simulink model "proyecto_automation"  (R2021a)
settings: Solver=VariableStepAuto  StartTime=0.0  StopTime=1900  RelTol=1e-3
values from neighbouring files (symbols this model uses):
  B = 0.029    [Parameters_setting.m]
  J = 0.1    [Parameters_setting.m]
  Ke = 0.6    [Parameters_setting.m]
  Kt = 0.6    [Parameters_setting.m]
  La = 1e-3    (= 0.001)    [Parameters_setting.m]
  Ra = 1    [Parameters_setting.m]
libraries: pid_lib x6, simulink x1
settings Model: Creator=csanc  LastModifiedBy=csanc

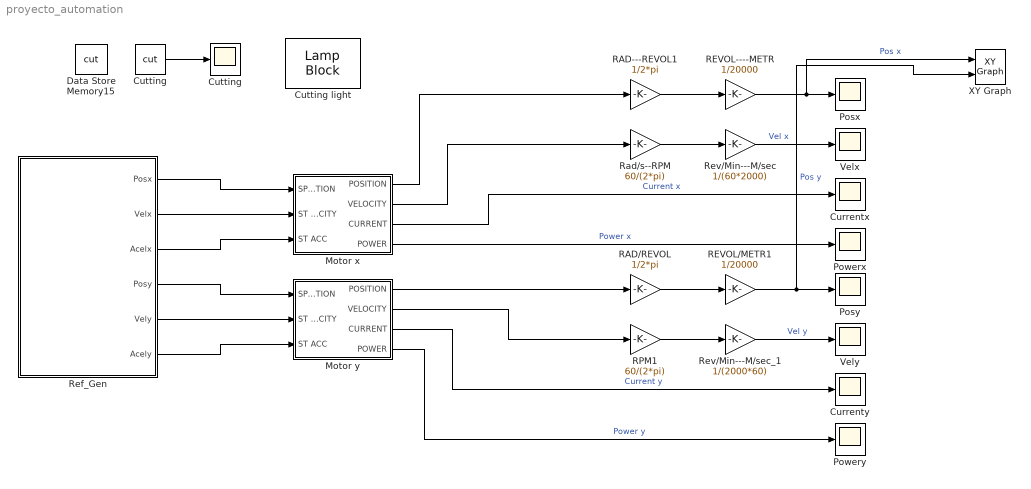
== system proyecto_automation ==
  Currentx : Scope
  Currenty : Scope
  Cutting : Scope
  "Cutting " : DataStoreRead  DataStoreName=cut  IndexOptions=Index vector (dialog)  Indices=1  OutputSizes=1
  Cutting light : LampBlock  Icon=LightingSwitch
  Data Store Memory15 : DataStoreMemory  DataStoreName=cut  ReadBeforeWriteMsg=warning  WriteAfterWriteMsg=warning  WriteAfterReadMsg=warning  ShowAdditionalParam=off
  Motor x : Subsystem
  Motor y : Subsystem
  Posx : Scope
  Posy : Scope
  Powerx : Scope
  Powery : Scope
  RAD---REVOL1 : Gain  Gain=1/2*pi
  RAD/REVOL : Gain  Gain=1/2*pi
  REVOL----METR : Gain  Gain=1/20000
  REVOL/METR1 : Gain  Gain=1/20000
  RPM1 : Gain  Gain=60/(2*pi)
  Rad/s--RPM : Gain  Gain=60/(2*pi)
  Ref_Gen : Subsystem
  Rev/Min---M/sec : Gain  Gain=1/(60*2000)
  Rev/Min---M/sec_1 : Gain  Gain=1/(2000*60)
  Velx : Scope
  Vely : Scope
  XY Graph : simulink/Sinks/XY Graph  xmin=0  xmax=3  ymin=0  ymax=2  st=1
  wires:
  Rad/s--RPM/1 -> Rev/Min---M/sec/1
  REVOL----METR/1 -> XY Graph/1, Posx/1  "Pos x"
  Rev/Min---M/sec/1 -> Velx/1  "Vel x"
  Ref_Gen/1(Posx) -> Motor x/1(SP POSITION)
  Ref_Gen/2(Velx) -> Motor x/2(ST VELOCITY)
  Ref_Gen/3(Acelx) -> Motor x/3(ST ACC)
  Motor x/2(VELOCITY) -> Rad/s--RPM/1
  Motor x/3(CURRENT) -> Currentx/1  "Current x"
  Motor x/4(POWER) -> Powerx/1  "Power x"
  Rev/Min---M/sec_1/1 -> Vely/1  "Vel y"
  REVOL/METR1/1 -> XY Graph/2, Posy/1  "Pos y"
  RAD/REVOL/1 -> REVOL/METR1/1
  RPM1/1 -> Rev/Min---M/sec_1/1
  Motor y/1(POSITION) -> RAD/REVOL/1
  Motor y/2(VELOCITY) -> RPM1/1
  Motor y/3(CURRENT) -> Currenty/1  "Current y"
  Motor y/4(POWER) -> Powery/1  "Power y"
  RAD---REVOL1/1 -> REVOL----METR/1
  Motor x/1(POSITION) -> RAD---REVOL1/1
  Ref_Gen/4(Posy) -> Motor y/1(SP POSITION)
  Ref_Gen/5(Vely) -> Motor y/2(ST VELOCITY)
  Ref_Gen/6(Acely) -> Motor y/3(ST ACC)
  "Cutting "/1 -> Cutting/1

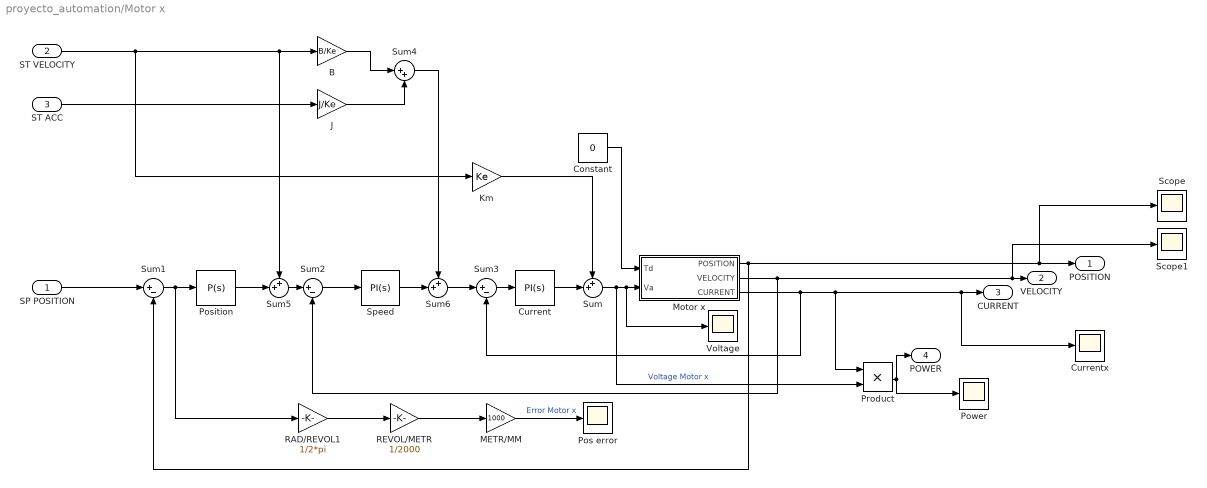
== system proyecto_automation/Motor x ==
  SP POSITION : Inport
  ST VELOCITY : Inport  Port=2
  ST ACC : Inport  Port=3
  B : Gain  Gain=B/Ke
  Constant : Constant  Value=0
  Current : pid_lib/PID Controller  Controller=PI  Form=Parallel  TimeDomain=Continuous-time  UseExternalTs=off  SampleTime=-1  IntegratorMethod=Forward Euler  FilterMethod=Forward Euler  ControllerParametersSource=internal  P=La*1000  I=Ra*1000  D=0  UseFilter=on  N=100  TunerSelectOption=Transfer Function Based (PID Tuner App)  InitialConditionSource=internal  InitialConditionForIntegrator=0  InitialConditionForFilter=0  DifferentiatorICPrevScaledInput=0  ExternalReset=none  TrackingMode=off  Kt=1  LimitOutput=off  SatLimitsSource=internal  UpperSaturationLimit=inf  LowerSaturationLimit=-inf  LinearizeAsGain=on  AntiWindupMode=none  Kb=1  POutMin=[]  POutMax=[]  IOutMin=[]  IOutMax=[]  DOutMin=[]  DOutMax=[]  NOutMin=[]  NOutMax=[]  SumOutMin=[]  SumOutMax=[]  SaturationOutMin=[]  SaturationOutMax=[]  PParamMin=[]  PParamMax=[]  IParamMin=[]  IParamMax=[]  DParamMin=[]  DParamMax=[]  NParamMin=[]  NParamMax=[]  KbParamMin=[]  KbParamMax=[]  KtParamMin=[]  KtParamMax=[]  KbOutMin=[]  KbOutMax=[]  KtOutMin=[]  KtOutMax=[]  IntegratorOutMin=[]  IntegratorOutMax=[]  FilterOutMin=[]  FilterOutMax=[]  SumI1OutMin=[]  SumI1OutMax=[]  SumI2OutMin=[]  SumI2OutMax=[]  SumI3OutMin=[]  SumI3OutMax=[]  SumI4OutMin=[]  SumI4OutMax=[]  SumDOutMin=[]  SumDOutMax=[]  DifferentiatorOutMin=[]  DifferentiatorOutMax=[]  FilterDiffOutCoefMin=[]  FilterDiffOutCoefMax=[]  ReciprocalOutMin=[]  ReciprocalOutMax=[]  SumDenOutMin=[]  SumDenOutMax=[]  SumNumOutMin=[]  SumNumOutMax=[]  DivideOutMin=[]  DivideOutMax=[]  UdiffTsProdOutMin=[]  UdiffTsProdOutMax=[]  NTsProdOutMin=[]  NTsProdOutMax=[]  UintegralTsProdOutMin=[]  UintegralTsProdOutMax=[]  UngainTsProdOutMin=[]  UngainTsProdOutMax=[]  IntegratorContinuousStateAttributes=''  IntegratorStateMustResolveToSignalObject=off  IntegratorRTWStateStorageClass=Auto  FilterContinuousStateAttributes=''  FilterStateMustResolveToSignalObject=off  FilterRTWStateStorageClass=Auto  ParallelPVariant=InternalParameters  IdealPVariant=Disabled  IVariant=InternalParameters  DVariant=Disabled  IntegratorVariant=Continuous  SatVariant=Disabled  AWVariant=Passthrough  PCopyVariant=Disabled  TRVariant=Disabled  FdbkBlocksVariant=Forward  IdealPFdbkVariant=Disabled  SatFdbkVariant=Disabled  DerivativeFilterVariant=Disabled  NVariant=Disabled  NCopyVariant=Disabled_SignalSpec  FilterICVariant=Disabled  IntegratorICVariant=InternalICs  ExternalResetVariant=Disabled  TRSumVariant=Passthrough  SumFdbkVariant=Disabled  SumVariant=Sum_PI  TsampFilterVariant=InternalTs  TsampNgainVariant=Passthrough  TsampIntegralVariant=Passthrough  ExternalSaturationOutDataTypeStr=Inherit: Same as second input
  Currentx : Scope
  J : Gain  Gain=J/Ke
  Km : Gain  Gain=Ke
  METR/MM : Gain  Gain=1000
  Motor x : Subsystem
  Pos error : Scope
  Position : pid_lib/PID Controller  Controller=P  Form=Parallel  TimeDomain=Continuous-time  UseExternalTs=on  SampleTime=-1  IntegratorMethod=Forward Euler  FilterMethod=Forward Euler  ControllerParametersSource=internal  P=1.1  I=1  D=0  UseFilter=on  N=100  TunerSelectOption=Transfer Function Based (PID Tuner App)  InitialConditionSource=internal  InitialConditionForIntegrator=0  InitialConditionForFilter=0  DifferentiatorICPrevScaledInput=0  ExternalReset=none  TrackingMode=off  Kt=1  LimitOutput=off  SatLimitsSource=internal  UpperSaturationLimit=inf  LowerSaturationLimit=-inf  LinearizeAsGain=on  AntiWindupMode=none  Kb=1  POutMin=[]  POutMax=[]  IOutMin=[]  IOutMax=[]  DOutMin=[]  DOutMax=[]  NOutMin=[]  NOutMax=[]  SumOutMin=[]  SumOutMax=[]  SaturationOutMin=[]  SaturationOutMax=[]  PParamMin=[]  PParamMax=[]  IParamMin=[]  IParamMax=[]  DParamMin=[]  DParamMax=[]  NParamMin=[]  NParamMax=[]  KbParamMin=[]  KbParamMax=[]  KtParamMin=[]  KtParamMax=[]  KbOutMin=[]  KbOutMax=[]  KtOutMin=[]  KtOutMax=[]  IntegratorOutMin=[]  IntegratorOutMax=[]  FilterOutMin=[]  FilterOutMax=[]  SumI1OutMin=[]  SumI1OutMax=[]  SumI2OutMin=[]  SumI2OutMax=[]  SumI3OutMin=[]  SumI3OutMax=[]  SumI4OutMin=[]  SumI4OutMax=[]  SumDOutMin=[]  SumDOutMax=[]  DifferentiatorOutMin=[]  DifferentiatorOutMax=[]  FilterDiffOutCoefMin=[]  FilterDiffOutCoefMax=[]  ReciprocalOutMin=[]  ReciprocalOutMax=[]  SumDenOutMin=[]  SumDenOutMax=[]  SumNumOutMin=[]  SumNumOutMax=[]  DivideOutMin=[]  DivideOutMax=[]  UdiffTsProdOutMin=[]  UdiffTsProdOutMax=[]  NTsProdOutMin=[]  NTsProdOutMax=[]  UintegralTsProdOutMin=[]  UintegralTsProdOutMax=[]  UngainTsProdOutMin=[]  UngainTsProdOutMax=[]  IntegratorContinuousStateAttributes=''  IntegratorStateMustResolveToSignalObject=off  IntegratorRTWStateStorageClass=Auto  FilterContinuousStateAttributes=''  FilterStateMustResolveToSignalObject=off  FilterRTWStateStorageClass=Auto  ParallelPVariant=InternalParameters  IdealPVariant=Disabled  IVariant=Disabled  DVariant=Disabled  IntegratorVariant=Disabled  SatVariant=Disabled  AWVariant=Disabled  PCopyVariant=Disabled  TRVariant=Disabled  FdbkBlocksVariant=Forward  IdealPFdbkVariant=Disabled  SatFdbkVariant=Disabled  DerivativeFilterVariant=Disabled  NVariant=Disabled  NCopyVariant=Disabled_SignalSpec  FilterICVariant=Disabled  IntegratorICVariant=Disabled  ExternalResetVariant=Disabled  TRSumVariant=Passthrough  SumFdbkVariant=Disabled  SumVariant=Passthrough_P  TsampFilterVariant=InternalTs  TsampNgainVariant=Passthrough  TsampIntegralVariant=Disabled_SignalSpec  ExternalSaturationOutDataTypeStr=Inherit: Same as second input
  Power : Scope
  Product : Product
  RAD/REVOL1 : Gain  Gain=1/2*pi
  REVOL/METR : Gain  Gain=1/2000
  Scope : Scope
  Scope1 : Scope
  Speed : pid_lib/PID Controller  Controller=PI  Form=Parallel  TimeDomain=Continuous-time  UseExternalTs=off  SampleTime=-1  IntegratorMethod=Forward Euler  FilterMethod=Forward Euler  ControllerParametersSource=internal  P=10*J  I=10*B  D=0  UseFilter=on  N=100  TunerSelectOption=Transfer Function Based (PID Tuner App)  InitialConditionSource=internal  InitialConditionForIntegrator=0  InitialConditionForFilter=0  DifferentiatorICPrevScaledInput=0  ExternalReset=none  TrackingMode=off  Kt=1  LimitOutput=off  SatLimitsSource=internal  UpperSaturationLimit=inf  LowerSaturationLimit=-inf  LinearizeAsGain=on  AntiWindupMode=none  Kb=1  POutMin=[]  POutMax=[]  IOutMin=[]  IOutMax=[]  DOutMin=[]  DOutMax=[]  NOutMin=[]  NOutMax=[]  SumOutMin=[]  SumOutMax=[]  SaturationOutMin=[]  SaturationOutMax=[]  PParamMin=[]  PParamMax=[]  IParamMin=[]  IParamMax=[]  DParamMin=[]  DParamMax=[]  NParamMin=[]  NParamMax=[]  KbParamMin=[]  KbParamMax=[]  KtParamMin=[]  KtParamMax=[]  KbOutMin=[]  KbOutMax=[]  KtOutMin=[]  KtOutMax=[]  IntegratorOutMin=[]  IntegratorOutMax=[]  FilterOutMin=[]  FilterOutMax=[]  SumI1OutMin=[]  SumI1OutMax=[]  SumI2OutMin=[]  SumI2OutMax=[]  SumI3OutMin=[]  SumI3OutMax=[]  SumI4OutMin=[]  SumI4OutMax=[]  SumDOutMin=[]  SumDOutMax=[]  DifferentiatorOutMin=[]  DifferentiatorOutMax=[]  FilterDiffOutCoefMin=[]  FilterDiffOutCoefMax=[]  ReciprocalOutMin=[]  ReciprocalOutMax=[]  SumDenOutMin=[]  SumDenOutMax=[]  SumNumOutMin=[]  SumNumOutMax=[]  DivideOutMin=[]  DivideOutMax=[]  UdiffTsProdOutMin=[]  UdiffTsProdOutMax=[]  NTsProdOutMin=[]  NTsProdOutMax=[]  UintegralTsProdOutMin=[]  UintegralTsProdOutMax=[]  UngainTsProdOutMin=[]  UngainTsProdOutMax=[]  IntegratorContinuousStateAttributes=''  IntegratorStateMustResolveToSignalObject=off  IntegratorRTWStateStorageClass=Auto  FilterContinuousStateAttributes=''  FilterStateMustResolveToSignalObject=off  FilterRTWStateStorageClass=Auto  ParallelPVariant=InternalParameters  IdealPVariant=Disabled  IVariant=InternalParameters  DVariant=Disabled  IntegratorVariant=Continuous  SatVariant=Disabled  AWVariant=Passthrough  PCopyVariant=Disabled  TRVariant=Disabled  FdbkBlocksVariant=Forward  IdealPFdbkVariant=Disabled  SatFdbkVariant=Disabled  DerivativeFilterVariant=Disabled  NVariant=Disabled  NCopyVariant=Disabled_SignalSpec  FilterICVariant=Disabled  IntegratorICVariant=InternalICs  ExternalResetVariant=Disabled  TRSumVariant=Passthrough  SumFdbkVariant=Disabled  SumVariant=Sum_PI  TsampFilterVariant=InternalTs  TsampNgainVariant=Passthrough  TsampIntegralVariant=Passthrough  ExternalSaturationOutDataTypeStr=Inherit: Same as second input
  Sum : Sum  Inputs=++|
  Sum1 : Sum  Inputs=|+-
  Sum2 : Sum  Inputs=|+-
  Sum3 : Sum  Inputs=|+-
  Sum4 : Sum  Inputs=|++
  Sum5 : Sum  Inputs=++|
  Sum6 : Sum  Inputs=++|
  Voltage : Scope
  POSITION : Outport
  VELOCITY : Outport  Port=2
  CURRENT : Outport  Port=3
  POWER : Outport  Port=4
  wires:
  Current/1 -> Sum/2
  ST VELOCITY/1 -> Km/1, Sum5/1, B/1
  Sum/1 -> Product/2, Voltage/1, Motor x/2(Va)  "Voltage Motor x"
  Sum2/1 -> Speed/1
  Motor x/2(VELOCITY) -> Sum2/2, Scope1/1, VELOCITY/1
  Motor x/3(CURRENT) -> Currentx/1, CURRENT/1, Product/1, Sum3/2
  J/1 -> Sum4/2
  Sum3/1 -> Current/1
  Sum1/1 -> RAD/REVOL1/1, Position/1
  ST ACC/1 -> J/1
  Motor x/1(POSITION) -> Scope/1, POSITION/1, Sum1/2
  Constant/1 -> Motor x/1(Td)
  B/1 -> Sum4/1
  Product/1 -> POWER/1, Power/1
  Position/1 -> Sum5/2
  Sum5/1 -> Sum2/1
  Sum6/1 -> Sum3/1
  Speed/1 -> Sum6/2
  SP POSITION/1 -> Sum1/1
  Km/1 -> Sum/1
  Sum4/1 -> Sum6/1
  RAD/REVOL1/1 -> REVOL/METR/1
  REVOL/METR/1 -> METR/MM/1
  METR/MM/1 -> Pos error/1  "Error Motor x"

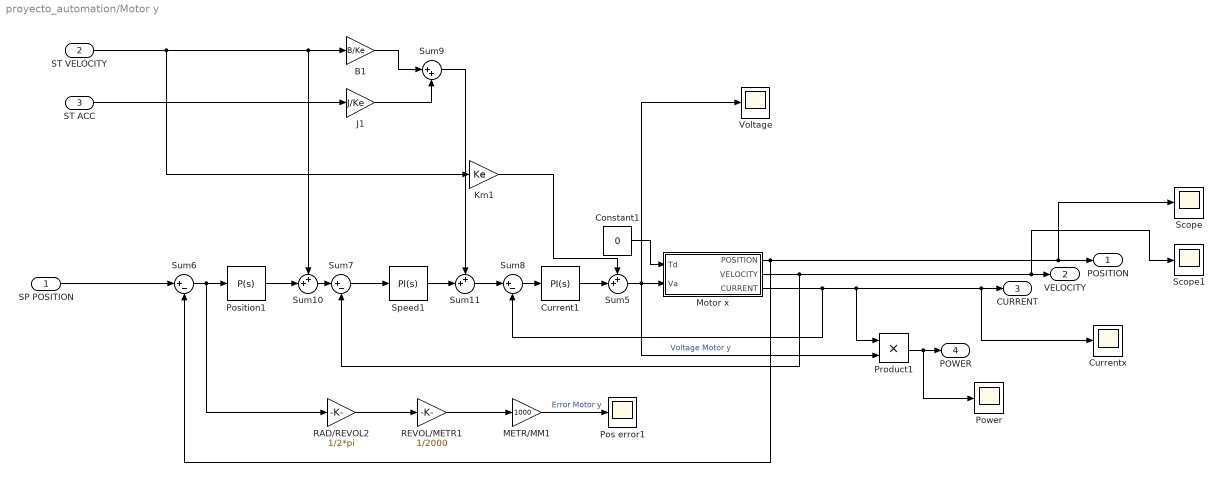
== system proyecto_automation/Motor y ==
  SP POSITION : Inport
  ST VELOCITY : Inport  Port=2
  ST ACC : Inport  Port=3
  B1 : Gain  Gain=B/Ke
  Constant1 : Constant  Value=0
  Current1 : pid_lib/PID Controller  Controller=PI  Form=Parallel  TimeDomain=Continuous-time  UseExternalTs=off  SampleTime=-1  IntegratorMethod=Forward Euler  FilterMethod=Forward Euler  ControllerParametersSource=internal  P=La*1000  I=Ra*1000  D=0  UseFilter=on  N=100  TunerSelectOption=Transfer Function Based (PID Tuner App)  InitialConditionSource=internal  InitialConditionForIntegrator=0  InitialConditionForFilter=0  DifferentiatorICPrevScaledInput=0  ExternalReset=none  TrackingMode=off  Kt=1  LimitOutput=off  SatLimitsSource=internal  UpperSaturationLimit=inf  LowerSaturationLimit=-inf  LinearizeAsGain=on  AntiWindupMode=none  Kb=1  POutMin=[]  POutMax=[]  IOutMin=[]  IOutMax=[]  DOutMin=[]  DOutMax=[]  NOutMin=[]  NOutMax=[]  SumOutMin=[]  SumOutMax=[]  SaturationOutMin=[]  SaturationOutMax=[]  PParamMin=[]  PParamMax=[]  IParamMin=[]  IParamMax=[]  DParamMin=[]  DParamMax=[]  NParamMin=[]  NParamMax=[]  KbParamMin=[]  KbParamMax=[]  KtParamMin=[]  KtParamMax=[]  KbOutMin=[]  KbOutMax=[]  KtOutMin=[]  KtOutMax=[]  IntegratorOutMin=[]  IntegratorOutMax=[]  FilterOutMin=[]  FilterOutMax=[]  SumI1OutMin=[]  SumI1OutMax=[]  SumI2OutMin=[]  SumI2OutMax=[]  SumI3OutMin=[]  SumI3OutMax=[]  SumI4OutMin=[]  SumI4OutMax=[]  SumDOutMin=[]  SumDOutMax=[]  DifferentiatorOutMin=[]  DifferentiatorOutMax=[]  FilterDiffOutCoefMin=[]  FilterDiffOutCoefMax=[]  ReciprocalOutMin=[]  ReciprocalOutMax=[]  SumDenOutMin=[]  SumDenOutMax=[]  SumNumOutMin=[]  SumNumOutMax=[]  DivideOutMin=[]  DivideOutMax=[]  UdiffTsProdOutMin=[]  UdiffTsProdOutMax=[]  NTsProdOutMin=[]  NTsProdOutMax=[]  UintegralTsProdOutMin=[]  UintegralTsProdOutMax=[]  UngainTsProdOutMin=[]  UngainTsProdOutMax=[]  IntegratorContinuousStateAttributes=''  IntegratorStateMustResolveToSignalObject=off  IntegratorRTWStateStorageClass=Auto  FilterContinuousStateAttributes=''  FilterStateMustResolveToSignalObject=off  FilterRTWStateStorageClass=Auto  ParallelPVariant=InternalParameters  IdealPVariant=Disabled  IVariant=InternalParameters  DVariant=Disabled  IntegratorVariant=Continuous  SatVariant=Disabled  AWVariant=Passthrough  PCopyVariant=Disabled  TRVariant=Disabled  FdbkBlocksVariant=Forward  IdealPFdbkVariant=Disabled  SatFdbkVariant=Disabled  DerivativeFilterVariant=Disabled  NVariant=Disabled  NCopyVariant=Disabled_SignalSpec  FilterICVariant=Disabled  IntegratorICVariant=InternalICs  ExternalResetVariant=Disabled  TRSumVariant=Passthrough  SumFdbkVariant=Disabled  SumVariant=Sum_PI  TsampFilterVariant=InternalTs  TsampNgainVariant=Passthrough  TsampIntegralVariant=Passthrough  ExternalSaturationOutDataTypeStr=Inherit: Same as second input
  Currentx : Scope
  J1 : Gain  Gain=J/Ke
  Km1 : Gain  Gain=Ke
  METR/MM1 : Gain  Gain=1000
  Motor x : Subsystem
  Pos error1 : Scope
  Position1 : pid_lib/PID Controller  Controller=P  Form=Parallel  TimeDomain=Continuous-time  UseExternalTs=on  SampleTime=-1  IntegratorMethod=Forward Euler  FilterMethod=Forward Euler  ControllerParametersSource=internal  P=1  I=1  D=0  UseFilter=on  N=100  TunerSelectOption=Transfer Function Based (PID Tuner App)  InitialConditionSource=internal  InitialConditionForIntegrator=0  InitialConditionForFilter=0  DifferentiatorICPrevScaledInput=0  ExternalReset=none  TrackingMode=off  Kt=1  LimitOutput=off  SatLimitsSource=internal  UpperSaturationLimit=inf  LowerSaturationLimit=-inf  LinearizeAsGain=on  AntiWindupMode=none  Kb=1  POutMin=[]  POutMax=[]  IOutMin=[]  IOutMax=[]  DOutMin=[]  DOutMax=[]  NOutMin=[]  NOutMax=[]  SumOutMin=[]  SumOutMax=[]  SaturationOutMin=[]  SaturationOutMax=[]  PParamMin=[]  PParamMax=[]  IParamMin=[]  IParamMax=[]  DParamMin=[]  DParamMax=[]  NParamMin=[]  NParamMax=[]  KbParamMin=[]  KbParamMax=[]  KtParamMin=[]  KtParamMax=[]  KbOutMin=[]  KbOutMax=[]  KtOutMin=[]  KtOutMax=[]  IntegratorOutMin=[]  IntegratorOutMax=[]  FilterOutMin=[]  FilterOutMax=[]  SumI1OutMin=[]  SumI1OutMax=[]  SumI2OutMin=[]  SumI2OutMax=[]  SumI3OutMin=[]  SumI3OutMax=[]  SumI4OutMin=[]  SumI4OutMax=[]  SumDOutMin=[]  SumDOutMax=[]  DifferentiatorOutMin=[]  DifferentiatorOutMax=[]  FilterDiffOutCoefMin=[]  FilterDiffOutCoefMax=[]  ReciprocalOutMin=[]  ReciprocalOutMax=[]  SumDenOutMin=[]  SumDenOutMax=[]  SumNumOutMin=[]  SumNumOutMax=[]  DivideOutMin=[]  DivideOutMax=[]  UdiffTsProdOutMin=[]  UdiffTsProdOutMax=[]  NTsProdOutMin=[]  NTsProdOutMax=[]  UintegralTsProdOutMin=[]  UintegralTsProdOutMax=[]  UngainTsProdOutMin=[]  UngainTsProdOutMax=[]  IntegratorContinuousStateAttributes=''  IntegratorStateMustResolveToSignalObject=off  IntegratorRTWStateStorageClass=Auto  FilterContinuousStateAttributes=''  FilterStateMustResolveToSignalObject=off  FilterRTWStateStorageClass=Auto  ParallelPVariant=InternalParameters  IdealPVariant=Disabled  IVariant=Disabled  DVariant=Disabled  IntegratorVariant=Disabled  SatVariant=Disabled  AWVariant=Disabled  PCopyVariant=Disabled  TRVariant=Disabled  FdbkBlocksVariant=Forward  IdealPFdbkVariant=Disabled  SatFdbkVariant=Disabled  DerivativeFilterVariant=Disabled  NVariant=Disabled  NCopyVariant=Disabled_SignalSpec  FilterICVariant=Disabled  IntegratorICVariant=Disabled  ExternalResetVariant=Disabled  TRSumVariant=Passthrough  SumFdbkVariant=Disabled  SumVariant=Passthrough_P  TsampFilterVariant=InternalTs  TsampNgainVariant=Passthrough  TsampIntegralVariant=Disabled_SignalSpec  ExternalSaturationOutDataTypeStr=Inherit: Same as second input
  Power : Scope
  Product1 : Product
  RAD/REVOL2 : Gain  Gain=1/2*pi
  REVOL/METR1 : Gain  Gain=1/2000
  Scope : Scope
  Scope1 : Scope
  Speed1 : pid_lib/PID Controller  Controller=PI  Form=Parallel  TimeDomain=Continuous-time  UseExternalTs=off  SampleTime=-1  IntegratorMethod=Forward Euler  FilterMethod=Forward Euler  ControllerParametersSource=internal  P=10*J  I=10*B  D=0  UseFilter=on  N=100  TunerSelectOption=Transfer Function Based (PID Tuner App)  InitialConditionSource=internal  InitialConditionForIntegrator=0  InitialConditionForFilter=0  DifferentiatorICPrevScaledInput=0  ExternalReset=none  TrackingMode=off  Kt=1  LimitOutput=off  SatLimitsSource=internal  UpperSaturationLimit=inf  LowerSaturationLimit=-inf  LinearizeAsGain=on  AntiWindupMode=none  Kb=1  POutMin=[]  POutMax=[]  IOutMin=[]  IOutMax=[]  DOutMin=[]  DOutMax=[]  NOutMin=[]  NOutMax=[]  SumOutMin=[]  SumOutMax=[]  SaturationOutMin=[]  SaturationOutMax=[]  PParamMin=[]  PParamMax=[]  IParamMin=[]  IParamMax=[]  DParamMin=[]  DParamMax=[]  NParamMin=[]  NParamMax=[]  KbParamMin=[]  KbParamMax=[]  KtParamMin=[]  KtParamMax=[]  KbOutMin=[]  KbOutMax=[]  KtOutMin=[]  KtOutMax=[]  IntegratorOutMin=[]  IntegratorOutMax=[]  FilterOutMin=[]  FilterOutMax=[]  SumI1OutMin=[]  SumI1OutMax=[]  SumI2OutMin=[]  SumI2OutMax=[]  SumI3OutMin=[]  SumI3OutMax=[]  SumI4OutMin=[]  SumI4OutMax=[]  SumDOutMin=[]  SumDOutMax=[]  DifferentiatorOutMin=[]  DifferentiatorOutMax=[]  FilterDiffOutCoefMin=[]  FilterDiffOutCoefMax=[]  ReciprocalOutMin=[]  ReciprocalOutMax=[]  SumDenOutMin=[]  SumDenOutMax=[]  SumNumOutMin=[]  SumNumOutMax=[]  DivideOutMin=[]  DivideOutMax=[]  UdiffTsProdOutMin=[]  UdiffTsProdOutMax=[]  NTsProdOutMin=[]  NTsProdOutMax=[]  UintegralTsProdOutMin=[]  UintegralTsProdOutMax=[]  UngainTsProdOutMin=[]  UngainTsProdOutMax=[]  IntegratorContinuousStateAttributes=''  IntegratorStateMustResolveToSignalObject=off  IntegratorRTWStateStorageClass=Auto  FilterContinuousStateAttributes=''  FilterStateMustResolveToSignalObject=off  FilterRTWStateStorageClass=Auto  ParallelPVariant=InternalParameters  IdealPVariant=Disabled  IVariant=InternalParameters  DVariant=Disabled  IntegratorVariant=Continuous  SatVariant=Disabled  AWVariant=Passthrough  PCopyVariant=Disabled  TRVariant=Disabled  FdbkBlocksVariant=Forward  IdealPFdbkVariant=Disabled  SatFdbkVariant=Disabled  DerivativeFilterVariant=Disabled  NVariant=Disabled  NCopyVariant=Disabled_SignalSpec  FilterICVariant=Disabled  IntegratorICVariant=InternalICs  ExternalResetVariant=Disabled  TRSumVariant=Passthrough  SumFdbkVariant=Disabled  SumVariant=Sum_PI  TsampFilterVariant=InternalTs  TsampNgainVariant=Passthrough  TsampIntegralVariant=Passthrough  ExternalSaturationOutDataTypeStr=Inherit: Same as second input
  Sum10 : Sum  Inputs=++|
  Sum11 : Sum  Inputs=++|
  Sum5 : Sum  Inputs=++|
  Sum6 : Sum  Inputs=|+-
  Sum7 : Sum  Inputs=|+-
  Sum8 : Sum  Inputs=|+-
  Sum9 : Sum  Inputs=|++
  Voltage : Scope
  POSITION : Outport
  VELOCITY : Outport  Port=2
  CURRENT : Outport  Port=3
  POWER : Outport  Port=4
  wires:
  RAD/REVOL2/1 -> REVOL/METR1/1
  Sum11/1 -> Sum8/1
  SP POSITION/1 -> Sum6/1
  Sum8/1 -> Current1/1
  Constant1/1 -> Motor x/1(Td)
  Sum9/1 -> Sum11/1
  Sum10/1 -> Sum7/1
  Speed1/1 -> Sum11/2
  Position1/1 -> Sum10/2
  B1/1 -> Sum9/1
  Km1/1 -> Sum5/1
  J1/1 -> Sum9/2
  Sum6/1 -> RAD/REVOL2/1, Position1/1
  Motor x/3(CURRENT) -> CURRENT/1, Currentx/1, Product1/1, Sum8/2
  Sum7/1 -> Speed1/1
  METR/MM1/1 -> Pos error1/1  "Error Motor y"
  REVOL/METR1/1 -> METR/MM1/1
  Sum5/1 -> Voltage/1, Product1/2, Motor x/2(Va)  "Voltage Motor y"
  Motor x/2(VELOCITY) -> Sum7/2, VELOCITY/1, Scope1/1
  ST VELOCITY/1 -> Km1/1, Sum10/1, B1/1
  Motor x/1(POSITION) -> POSITION/1, Scope/1, Sum6/2
  ST ACC/1 -> J1/1
  Current1/1 -> Sum5/2
  Product1/1 -> Power/1, POWER/1

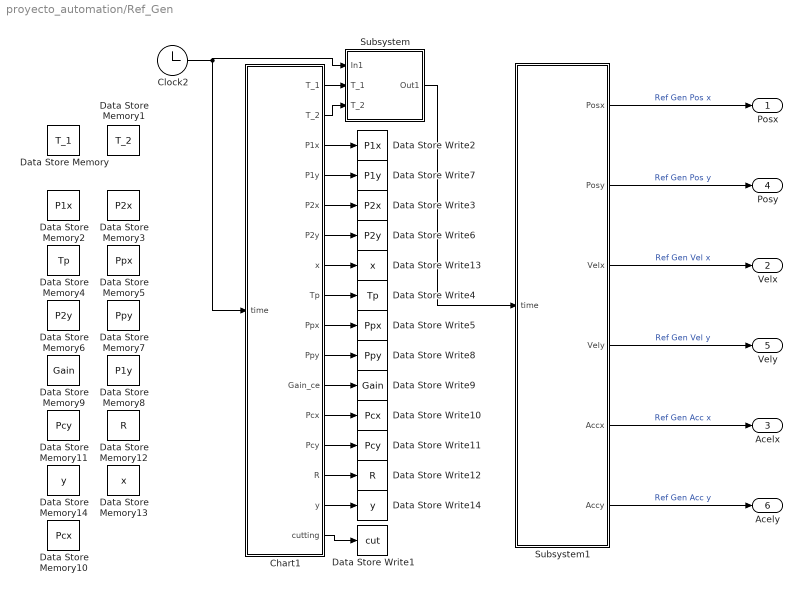
== system proyecto_automation/Ref_Gen ==
  Chart1 : Stateflow chart  TreatAsAtomicUnit=on
  Clock2 : Clock
  Data Store Memory : DataStoreMemory  DataStoreName=T_1  ReadBeforeWriteMsg=warning  WriteAfterWriteMsg=warning  WriteAfterReadMsg=warning  ShowAdditionalParam=off
  Data Store Memory1 : DataStoreMemory  DataStoreName=T_2  ReadBeforeWriteMsg=warning  WriteAfterWriteMsg=warning  WriteAfterReadMsg=warning  ShowAdditionalParam=off
  Data Store Memory10 : DataStoreMemory  DataStoreName=Pcx  ReadBeforeWriteMsg=warning  WriteAfterWriteMsg=warning  WriteAfterReadMsg=warning  ShowAdditionalParam=off
  Data Store Memory11 : DataStoreMemory  DataStoreName=Pcy  ReadBeforeWriteMsg=warning  WriteAfterWriteMsg=warning  WriteAfterReadMsg=warning  ShowAdditionalParam=off
  Data Store Memory12 : DataStoreMemory  DataStoreName=R  ReadBeforeWriteMsg=warning  WriteAfterWriteMsg=warning  WriteAfterReadMsg=warning  ShowAdditionalParam=off
  Data Store Memory13 : DataStoreMemory  DataStoreName=x  ReadBeforeWriteMsg=warning  WriteAfterWriteMsg=warning  WriteAfterReadMsg=warning  ShowAdditionalParam=off
  Data Store Memory14 : DataStoreMemory  DataStoreName=y  ReadBeforeWriteMsg=warning  WriteAfterWriteMsg=warning  WriteAfterReadMsg=warning  ShowAdditionalParam=off
  Data Store Memory2 : DataStoreMemory  DataStoreName=P1x  ReadBeforeWriteMsg=warning  WriteAfterWriteMsg=warning  WriteAfterReadMsg=warning  ShowAdditionalParam=off
  Data Store Memory3 : DataStoreMemory  DataStoreName=P2x  ReadBeforeWriteMsg=warning  WriteAfterWriteMsg=warning  WriteAfterReadMsg=warning  ShowAdditionalParam=off
  Data Store Memory4 : DataStoreMemory  DataStoreName=Tp  ReadBeforeWriteMsg=warning  WriteAfterWriteMsg=warning  WriteAfterReadMsg=warning  ShowAdditionalParam=off
  Data Store Memory5 : DataStoreMemory  DataStoreName=Ppx  ReadBeforeWriteMsg=warning  WriteAfterWriteMsg=warning  WriteAfterReadMsg=warning  ShowAdditionalParam=off
  Data Store Memory6 : DataStoreMemory  DataStoreName=P2y  ReadBeforeWriteMsg=warning  WriteAfterWriteMsg=warning  WriteAfterReadMsg=warning  ShowAdditionalParam=off
  Data Store Memory7 : DataStoreMemory  DataStoreName=Ppy  ReadBeforeWriteMsg=warning  WriteAfterWriteMsg=warning  WriteAfterReadMsg=warning  ShowAdditionalParam=off
  Data Store Memory8 : DataStoreMemory  DataStoreName=P1y  ReadBeforeWriteMsg=warning  WriteAfterWriteMsg=warning  WriteAfterReadMsg=warning  ShowAdditionalParam=off
  Data Store Memory9 : DataStoreMemory  DataStoreName=Gain  ReadBeforeWriteMsg=warning  WriteAfterWriteMsg=warning  WriteAfterReadMsg=warning  ShowAdditionalParam=off
  Data Store Write1 : DataStoreWrite  DataStoreName=cut  IndexOptions=Index vector (dialog)  Indices=1  OutputSizes=1
  Data Store Write10 : DataStoreWrite  DataStoreName=Pcx  IndexOptions=Index vector (dialog)  Indices=1  OutputSizes=1
  Data Store Write11 : DataStoreWrite  DataStoreName=Pcy  IndexOptions=Index vector (dialog)  Indices=1  OutputSizes=1
  Data Store Write12 : DataStoreWrite  DataStoreName=R  IndexOptions=Index vector (dialog)  Indices=1  OutputSizes=1
  Data Store Write13 : DataStoreWrite  DataStoreName=x  IndexOptions=Index vector (dialog)  Indices=1  OutputSizes=1
  Data Store Write14 : DataStoreWrite  DataStoreName=y  IndexOptions=Index vector (dialog)  Indices=1  OutputSizes=1
  Data Store Write2 : DataStoreWrite  DataStoreName=P1x  IndexOptions=Index vector (dialog)  Indices=1  OutputSizes=1
  Data Store Write3 : DataStoreWrite  DataStoreName=P2x  IndexOptions=Index vector (dialog)  Indices=1  OutputSizes=1
  Data Store Write4 : DataStoreWrite  DataStoreName=Tp  IndexOptions=Index vector (dialog)  Indices=1  OutputSizes=1
  Data Store Write5 : DataStoreWrite  DataStoreName=Ppx  IndexOptions=Index vector (dialog)  Indices=1  OutputSizes=1
  Data Store Write6 : DataStoreWrite  DataStoreName=P2y  IndexOptions=Index vector (dialog)  Indices=1  OutputSizes=1
  Data Store Write7 : DataStoreWrite  DataStoreName=P1y  IndexOptions=Index vector (dialog)  Indices=1  OutputSizes=1
  Data Store Write8 : DataStoreWrite  DataStoreName=Ppy  IndexOptions=Index vector (dialog)  Indices=1  OutputSizes=1
  Data Store Write9 : DataStoreWrite  DataStoreName=Gain  IndexOptions=Index vector (dialog)  Indices=1  OutputSizes=1
  Subsystem : Subsystem
  Subsystem1 : Subsystem
  Posx : Outport
  Velx : Outport  Port=2
  Acelx : Outport  Port=3
  Posy : Outport  Port=4
  Vely : Outport  Port=5
  Acely : Outport  Port=6
  wires:
  Chart1/1(T_1) -> Subsystem/2(T_1)
  Chart1/2(T_2) -> Subsystem/3(T_2)
  Chart1/3(P1x) -> Data Store Write2/1
  Chart1/5(P2x) -> Data Store Write3/1
  Chart1/8(Tp) -> Data Store Write4/1
  Chart1/9(Ppx) -> Data Store Write5/1
  Chart1/6(P2y) -> Data Store Write6/1
  Chart1/4(P1y) -> Data Store Write7/1
  Chart1/10(Ppy) -> Data Store Write8/1
  Chart1/11(Gain_ce) -> Data Store Write9/1
  Chart1/12(Pcx) -> Data Store Write10/1
  Chart1/13(Pcy) -> Data Store Write11/1
  Chart1/14(R) -> Data Store Write12/1
  Chart1/7(x) -> Data Store Write13/1
  Chart1/15(y) -> Data Store Write14/1
  Subsystem/1(Out1) -> Subsystem1/1(time)
  Clock2/1 -> Subsystem/1(In1), Chart1/1(time)
  Subsystem1/1(Posx) -> Posx/1  "Ref Gen Pos x"
  Subsystem1/2(Posy) -> Posy/1  "Ref Gen Pos y"
  Subsystem1/3(Velx) -> Velx/1  "Ref Gen Vel x"
  Subsystem1/4(Vely) -> Vely/1  "Ref Gen Vel y"
  Subsystem1/5(Accx) -> Acelx/1  "Ref Gen Acc x"
  Subsystem1/6(Accy) -> Acely/1  "Ref Gen Acc y"
  Chart1/16(cutting) -> Data Store Write1/1

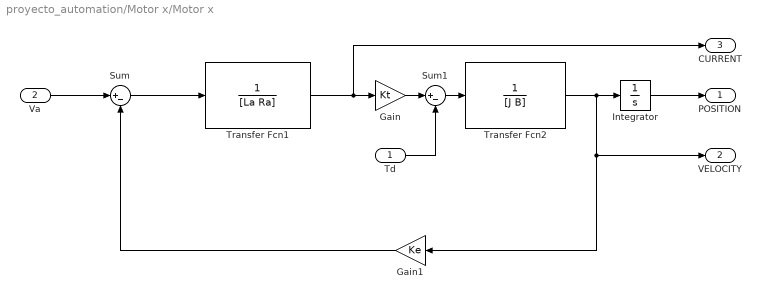
== system proyecto_automation/Motor x/Motor x ==
  Td : Inport
  Va : Inport  Port=2
  Gain : Gain  Gain=Kt
  Gain1 : Gain  Gain=Ke
  Integrator : Integrator
  Sum : Sum  Inputs=|+-
  Sum1 : Sum  Inputs=|+-
  Transfer Fcn1 : TransferFcn  Denominator=[La Ra]
  Transfer Fcn2 : TransferFcn  Denominator=[J B]
  POSITION : Outport
  VELOCITY : Outport  Port=2
  CURRENT : Outport  Port=3
  wires:
  Transfer Fcn1/1 -> CURRENT/1, Gain/1
  Integrator/1 -> POSITION/1
  Transfer Fcn2/1 -> Gain1/1, VELOCITY/1, Integrator/1
  Va/1 -> Sum/1
  Sum/1 -> Transfer Fcn1/1
  Gain1/1 -> Sum/2
  Gain/1 -> Sum1/1
  Sum1/1 -> Transfer Fcn2/1
  Td/1 -> Sum1/2

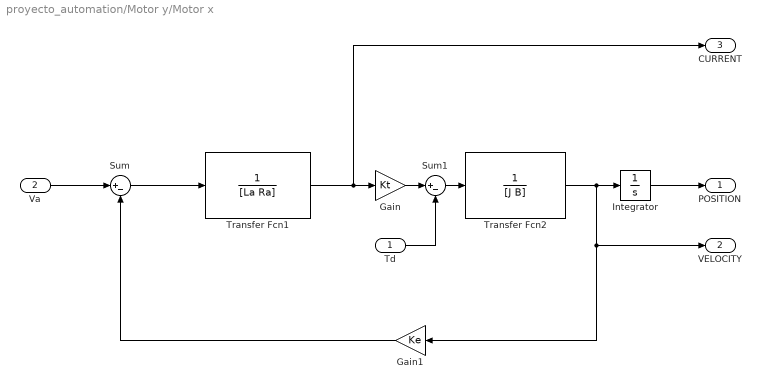
== system proyecto_automation/Motor y/Motor x ==
  Td : Inport
  Va : Inport  Port=2
  Gain : Gain  Gain=Kt
  Gain1 : Gain  Gain=Ke
  Integrator : Integrator
  Sum : Sum  Inputs=|+-
  Sum1 : Sum  Inputs=|+-
  Transfer Fcn1 : TransferFcn  Denominator=[La Ra]
  Transfer Fcn2 : TransferFcn  Denominator=[J B]
  POSITION : Outport
  VELOCITY : Outport  Port=2
  CURRENT : Outport  Port=3
  wires:
  Transfer Fcn1/1 -> CURRENT/1, Gain/1
  Integrator/1 -> POSITION/1
  Transfer Fcn2/1 -> Gain1/1, VELOCITY/1, Integrator/1
  Va/1 -> Sum/1
  Sum/1 -> Transfer Fcn1/1
  Gain1/1 -> Sum/2
  Gain/1 -> Sum1/1
  Sum1/1 -> Transfer Fcn2/1
  Td/1 -> Sum1/2

== system proyecto_automation/Ref_Gen/Subsystem ==
  In1 : Inport
  T_1 : Inport  Port=2
  T_2 : Inport  Port=3
  Add7 : Sum  Inputs=+-
  Add8 : Sum  Inputs=+-
  Add9 : Sum  Inputs=+-
  Constant21 : Constant  Value=0
  Constant25 : Constant  Value=0
  Scope : Scope
  Switch7 : Switch  Criteria=u2 > Threshold
  Switch9 : Switch  Criteria=u2 > Threshold
  Out1 : Outport
  wires:
  In1/1 -> Add7/1, Add8/1
  Switch9/1 -> Add9/2
  Constant25/1 -> Switch9/3
  Add7/1 -> Switch7/1, Switch7/2
  Add8/1 -> Switch9/1, Switch9/2
  Switch7/1 -> Add9/1
  T_2/1 -> Add8/2
  Constant21/1 -> Switch7/3
  Add9/1 -> Scope/1, Out1/1
  T_1/1 -> Add7/2

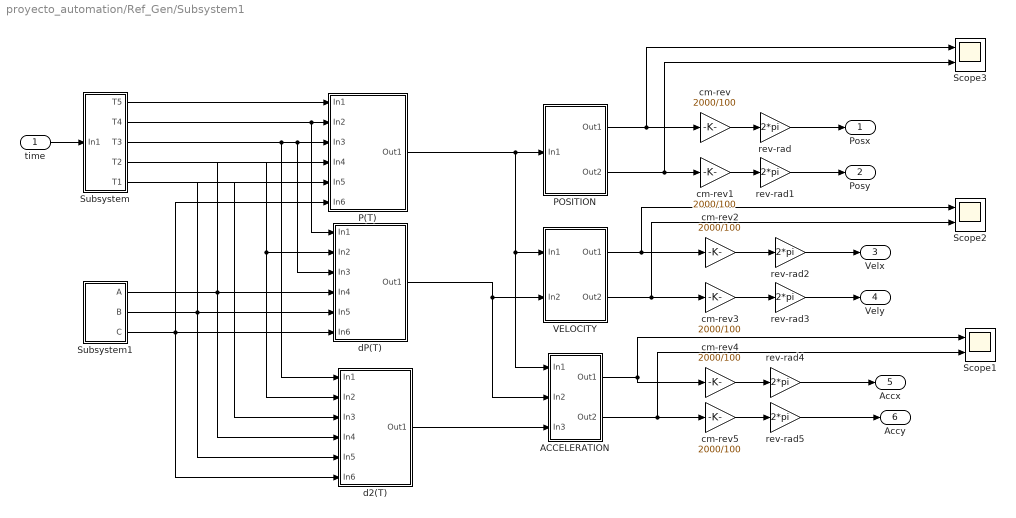
== system proyecto_automation/Ref_Gen/Subsystem1 ==
  time : Inport
  ACCELERATION : Subsystem
  P(T) : Subsystem
  POSITION : Subsystem
  Scope1 : Scope  NumInputPorts=2
  Scope2 : Scope  NumInputPorts=2
  Scope3 : Scope  NumInputPorts=2
  Subsystem : Subsystem
  Subsystem1 : Subsystem
  VELOCITY : Subsystem
  cm-rev{,1..5} (6 alike) : Gain  Gain=2000/100
  d2(T) : Subsystem
  dP(T) : Subsystem
  rev-rad{,1..5} (6 alike) : Gain  Gain=2*pi
  Posx : Outport
  Posy : Outport  Port=2
  Velx : Outport  Port=3
  Vely : Outport  Port=4
  Accx : Outport  Port=5
  Accy : Outport  Port=6
  wires:
  cm-rev/1 -> rev-rad/1
  cm-rev1/1 -> rev-rad1/1
  rev-rad/1 -> Posx/1
  rev-rad1/1 -> Posy/1
  cm-rev2/1 -> rev-rad2/1
  rev-rad2/1 -> Velx/1
  rev-rad3/1 -> Vely/1
  cm-rev3/1 -> rev-rad3/1
  rev-rad4/1 -> Accx/1
  cm-rev4/1 -> rev-rad4/1
  rev-rad5/1 -> Accy/1
  cm-rev5/1 -> rev-rad5/1
  time/1 -> Subsystem/1(In1)
  Subsystem/1(T5) -> P(T)/1(In1)
  Subsystem/2(T4) -> dP(T)/1(In1), P(T)/2(In2)
  Subsystem/3(T3) -> P(T)/3(In3), dP(T)/3(In3), d2(T)/1(In1)
  Subsystem1/1(A) -> d2(T)/4(In4), dP(T)/4(In4), P(T)/4(In4)
  Subsystem1/2(B) -> dP(T)/5(In5), P(T)/5(In5), d2(T)/5(In5)
  Subsystem1/3(C) -> d2(T)/6(In6), dP(T)/6(In6), P(T)/6(In6)
  Subsystem/4(T2) -> dP(T)/2(In2), d2(T)/2(In2)
  Subsystem/5(T1) -> d2(T)/3(In3)
  POSITION/2(Out2) -> Scope3/2, cm-rev1/1
  POSITION/1(Out1) -> Scope3/1, cm-rev/1
  P(T)/1(Out1) -> ACCELERATION/1(In1), VELOCITY/1(In1), POSITION/1(In1)
  VELOCITY/2(Out2) -> Scope2/2, cm-rev3/1
  dP(T)/1(Out1) -> ACCELERATION/2(In2), VELOCITY/2(In2)
  ACCELERATION/2(Out2) -> Scope1/2, cm-rev5/1
  d2(T)/1(Out1) -> ACCELERATION/3(In3)
  ACCELERATION/1(Out1) -> Scope1/1, cm-rev4/1
  VELOCITY/1(Out1) -> Scope2/1, cm-rev2/1

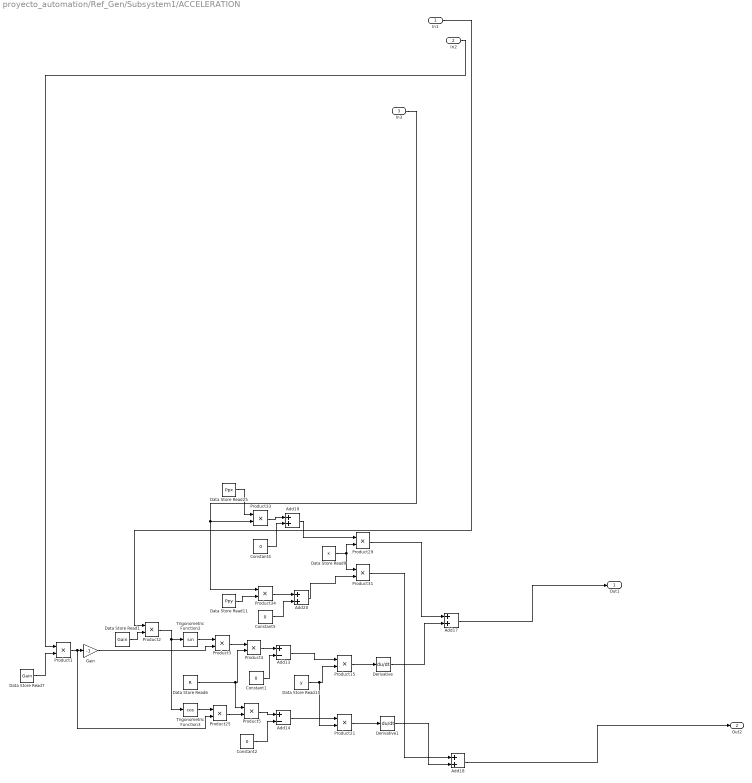
== system proyecto_automation/Ref_Gen/Subsystem1/ACCELERATION ==
  In1 : Inport
  In2 : Inport  Port=2
  In3 : Inport  Port=3
  Add13 : Sum  Inputs=+-
  Add14 : Sum  Inputs=+-
  Add{17..20} (4 alike) : Sum
  Constant{1..2,4..5} (4 alike) : Constant  Value=0
  Data Store Read1 : DataStoreRead  DataStoreName=Gain  IndexOptions=Index vector (dialog)  Indices=1  OutputSizes=1
  Data Store Read10 : DataStoreRead  DataStoreName=y  IndexOptions=Index vector (dialog)  Indices=1  OutputSizes=1
  Data Store Read11 : DataStoreRead  DataStoreName=Ppy  IndexOptions=Index vector (dialog)  Indices=1  OutputSizes=1
  Data Store Read25 : DataStoreRead  DataStoreName=Ppx  IndexOptions=Index vector (dialog)  Indices=1  OutputSizes=1
  Data Store Read6 : DataStoreRead  DataStoreName=R  IndexOptions=Index vector (dialog)  Indices=1  OutputSizes=1
  Data Store Read7 : DataStoreRead  DataStoreName=Gain  IndexOptions=Index vector (dialog)  Indices=1  OutputSizes=1
  Data Store Read9 : DataStoreRead  DataStoreName=x  IndexOptions=Index vector (dialog)  Indices=1  OutputSizes=1
  Derivative : Derivative
  Derivative1 : Derivative
  Gain : Gain  Gain=-1
  Product{1..5,15,21,25,29,31,33..34} (12 alike) : Product
  Trigonometric Function2 : Trigonometry
  Trigonometric Function3 : Trigonometry  Operator=cos
  Out1 : Outport
  Out2 : Outport  Port=2
  wires:
  In3/1 -> Product34/1, Product33/2
  Trigonometric Function2/1 -> Product3/1
  Product21/1 -> Derivative1/1
  Add13/1 -> Product15/1
  Data Store Read1/1 -> Product2/2
  Trigonometric Function3/1 -> Product25/1
  Product4/1 -> Add13/1
  Data Store Read25/1 -> Product33/1
  Constant4/1 -> Add19/2
  In1/1 -> Product2/1
  Constant2/1 -> Add14/2
  Add17/1 -> Out1/1
  Product5/1 -> Add14/1
  Product25/1 -> Product5/2
  Gain/1 -> Product3/2
  Product1/1 -> Product25/2, Gain/1
  Data Store Read6/1 -> Product5/1, Product4/2
  Data Store Read11/1 -> Product34/2
  In2/1 -> Product1/1
  Add20/1 -> Product31/2
  Data Store Read7/1 -> Product1/2
  Data Store Read10/1 -> Product21/2, Product15/2
  Derivative1/1 -> Add18/2
  Product2/1 -> Trigonometric Function3/1, Trigonometric Function2/1
  Product31/1 -> Add18/1
  Add14/1 -> Product21/1
  Product3/1 -> Product4/1
  Product33/1 -> Add19/1
  Product15/1 -> Derivative/1
  Derivative/1 -> Add17/2
  Product29/1 -> Add17/1
  Add19/1 -> Product29/1
  Product34/1 -> Add20/1
  Data Store Read9/1 -> Product31/1, Product29/2
  Constant5/1 -> Add20/2
  Add18/1 -> Out2/1
  Constant1/1 -> Add13/2

== system proyecto_automation/Ref_Gen/Subsystem1/P(T) ==
  In1 : Inport
  In2 : Inport  Port=2
  In3 : Inport  Port=3
  In4 : Inport  Port=4
  In5 : Inport  Port=5
  In6 : Inport  Port=6
  Add21 : Sum  Inputs=+++
  Product39 : Product
  Product40 : Product
  Product41 : Product
  Out1 : Outport
  wires:
  Product41/1 -> Add21/2
  In1/1 -> Product40/1
  In3/1 -> Product39/1
  In6/1 -> Product39/2
  Product40/1 -> Add21/1
  Product39/1 -> Add21/3
  In2/1 -> Product41/1
  In5/1 -> Product41/2
  Add21/1 -> Out1/1
  In4/1 -> Product40/2

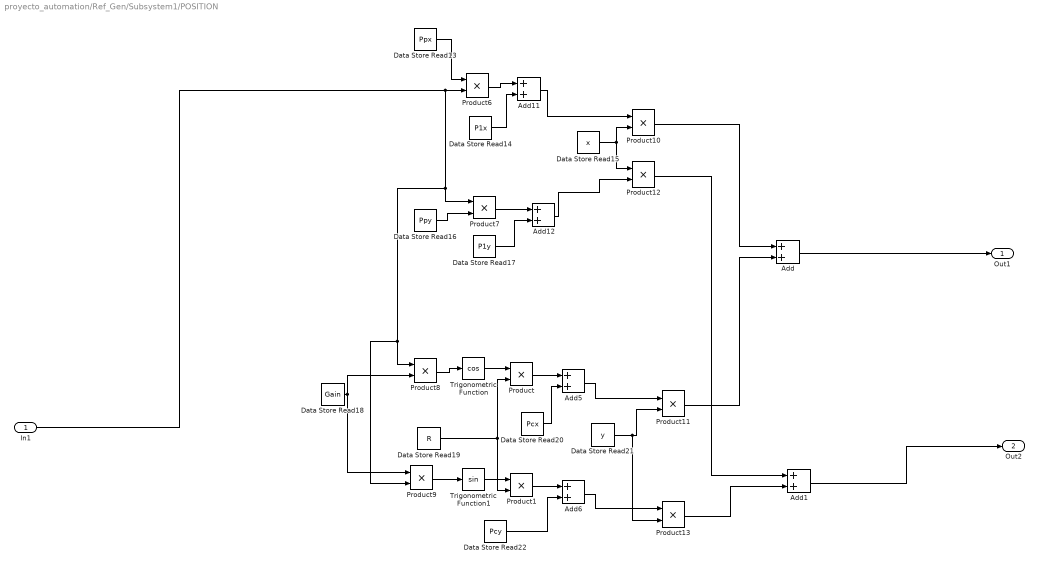
== system proyecto_automation/Ref_Gen/Subsystem1/POSITION ==
  In1 : Inport
  Add{,1,5..6,11..12} (6 alike) : Sum
  Data Store Read13 : DataStoreRead  DataStoreName=Ppx  IndexOptions=Index vector (dialog)  Indices=1  OutputSizes=1
  Data Store Read14 : DataStoreRead  DataStoreName=P1x  IndexOptions=Index vector (dialog)  Indices=1  OutputSizes=1
  Data Store Read15 : DataStoreRead  DataStoreName=x  IndexOptions=Index vector (dialog)  Indices=1  OutputSizes=1
  Data Store Read16 : DataStoreRead  DataStoreName=Ppy  IndexOptions=Index vector (dialog)  Indices=1  OutputSizes=1
  Data Store Read17 : DataStoreRead  DataStoreName=P1y  IndexOptions=Index vector (dialog)  Indices=1  OutputSizes=1
  Data Store Read18 : DataStoreRead  DataStoreName=Gain  IndexOptions=Index vector (dialog)  Indices=1  OutputSizes=1
  Data Store Read19 : DataStoreRead  DataStoreName=R  IndexOptions=Index vector (dialog)  Indices=1  OutputSizes=1
  Data Store Read20 : DataStoreRead  DataStoreName=Pcx  IndexOptions=Index vector (dialog)  Indices=1  OutputSizes=1
  Data Store Read21 : DataStoreRead  DataStoreName=y  IndexOptions=Index vector (dialog)  Indices=1  OutputSizes=1
  Data Store Read22 : DataStoreRead  DataStoreName=Pcy  IndexOptions=Index vector (dialog)  Indices=1  OutputSizes=1
  Product{,1,6..13} (10 alike) : Product
  Trigonometric Function : Trigonometry  Operator=cos
  Trigonometric Function1 : Trigonometry
  Out1 : Outport
  Out2 : Outport  Port=2
  wires:
  Data Store Read14/1 -> Add11/2
  Add6/1 -> Product13/1
  Data Store Read21/1 -> Product13/2, Product11/2
  Data Store Read17/1 -> Add12/2
  Data Store Read16/1 -> Product7/2
  Add11/1 -> Product10/1
  Data Store Read22/1 -> Add6/2
  Product6/1 -> Add11/1
  Product8/1 -> Trigonometric Function/1
  In1/1 -> Product6/2, Product7/1, Product9/2, Product8/1
  Product7/1 -> Add12/1
  Data Store Read18/1 -> Product8/2, Product9/1
  Trigonometric Function1/1 -> Product1/1
  Data Store Read19/1 -> Product1/2, Product/2
  Add5/1 -> Product11/1
  Data Store Read20/1 -> Add5/2
  Product/1 -> Add5/1
  Data Store Read13/1 -> Product6/1
  Product1/1 -> Add6/1
  Product11/1 -> Add/2
  Data Store Read15/1 -> Product12/1, Product10/2
  Trigonometric Function/1 -> Product/1
  Product13/1 -> Add1/2
  Product12/1 -> Add1/1
  Product9/1 -> Trigonometric Function1/1
  Product10/1 -> Add/1
  Add1/1 -> Out2/1
  Add12/1 -> Product12/2
  Add/1 -> Out1/1

== system proyecto_automation/Ref_Gen/Subsystem1/Subsystem ==
  In1 : Inport
  t{2..5} (4 alike) : Product
  T5 : Outport
  T4 : Outport  Port=2
  T3 : Outport  Port=3
  T2 : Outport  Port=4
  T1 : Outport  Port=5
  wires:
  t4/1 -> T4/1, t5/2
  t3/1 -> T3/1, t4/2
  t2/1 -> T2/1, t3/2
  t5/1 -> T5/1
  In1/1 -> t2/1, t3/1, t5/1, t4/1, T1/1, t2/2

== system proyecto_automation/Ref_Gen/Subsystem1/Subsystem1 ==
  Data Store Read1 : DataStoreRead  DataStoreName=Tp  IndexOptions=Index vector (dialog)  Indices=1  OutputSizes=1
  Math Reciprocal1 : Math  Operator=reciprocal  SignedPower=on  SaturateOnIntegerOverflow=on
  a : Subsystem
  b : Subsystem
  c : Subsystem
  A : Outport
  B : Outport  Port=2
  C : Outport  Port=3
  wires:
  Data Store Read1/1 -> Math Reciprocal1/1
  Math Reciprocal1/1 -> b/1(In1), a/1(In1), c/1(In1)
  a/1(Out1) -> A/1
  c/1(Out1) -> C/1
  b/1(Out1) -> B/1

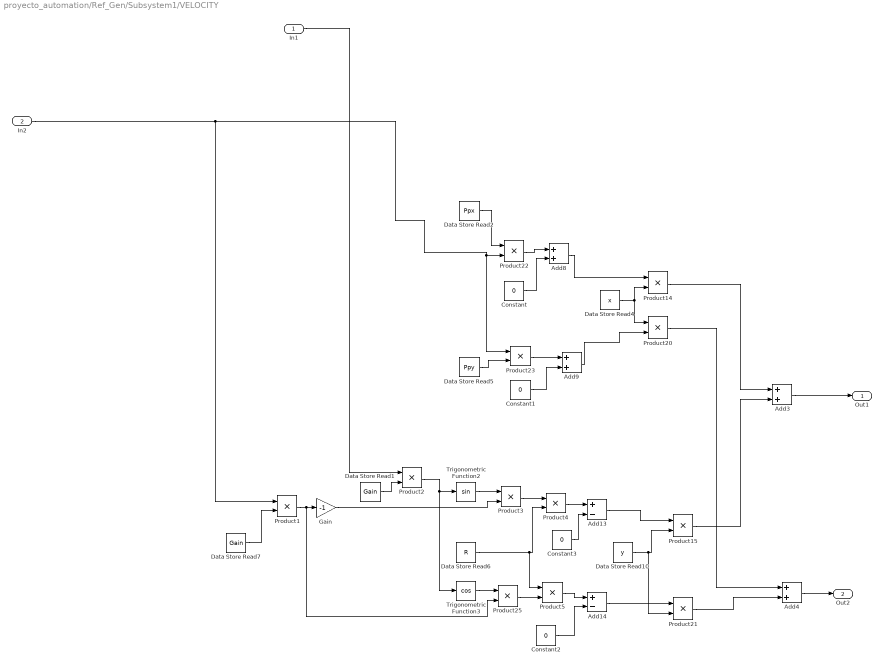
== system proyecto_automation/Ref_Gen/Subsystem1/VELOCITY ==
  In1 : Inport
  In2 : Inport  Port=2
  Add13 : Sum  Inputs=+-
  Add14 : Sum  Inputs=+-
  Add{3..4,8..9} (4 alike) : Sum
  Constant{,1..3} (4 alike) : Constant  Value=0
  Data Store Read1 : DataStoreRead  DataStoreName=Gain  IndexOptions=Index vector (dialog)  Indices=1  OutputSizes=1
  Data Store Read10 : DataStoreRead  DataStoreName=y  IndexOptions=Index vector (dialog)  Indices=1  OutputSizes=1
  Data Store Read2 : DataStoreRead  DataStoreName=Ppx  IndexOptions=Index vector (dialog)  Indices=1  OutputSizes=1
  Data Store Read4 : DataStoreRead  DataStoreName=x  IndexOptions=Index vector (dialog)  Indices=1  OutputSizes=1
  Data Store Read5 : DataStoreRead  DataStoreName=Ppy  IndexOptions=Index vector (dialog)  Indices=1  OutputSizes=1
  Data Store Read6 : DataStoreRead  DataStoreName=R  IndexOptions=Index vector (dialog)  Indices=1  OutputSizes=1
  Data Store Read7 : DataStoreRead  DataStoreName=Gain  IndexOptions=Index vector (dialog)  Indices=1  OutputSizes=1
  Gain : Gain  Gain=-1
  Product{1..5,14..15,20..23,25} (12 alike) : Product
  Trigonometric Function2 : Trigonometry
  Trigonometric Function3 : Trigonometry  Operator=cos
  Out1 : Outport
  Out2 : Outport  Port=2
  wires:
  Data Store Read4/1 -> Product20/1, Product14/2
  Trigonometric Function2/1 -> Product3/1
  Product1/1 -> Product25/2, Gain/1
  Data Store Read10/1 -> Product21/2, Product15/2
  Add14/1 -> Product21/1
  Product2/1 -> Trigonometric Function3/1, Trigonometric Function2/1
  Product3/1 -> Product4/1
  In2/1 -> Product1/1, Product22/2, Product23/1
  Data Store Read7/1 -> Product1/2
  Data Store Read6/1 -> Product5/1, Product4/2
  Product23/1 -> Add9/1
  Product5/1 -> Add14/1
  Add8/1 -> Product14/1
  Product25/1 -> Product5/2
  Constant/1 -> Add8/2
  Add9/1 -> Product20/2
  Product20/1 -> Add4/1
  Add13/1 -> Product15/1
  Data Store Read2/1 -> Product22/1
  Constant1/1 -> Add9/2
  Data Store Read5/1 -> Product23/2
  Gain/1 -> Product3/2
  Product15/1 -> Add3/2
  Product21/1 -> Add4/2
  Add3/1 -> Out1/1
  Product14/1 -> Add3/1
  Constant2/1 -> Add14/2
  Product4/1 -> Add13/1
  In1/1 -> Product2/1
  Product22/1 -> Add8/1
  Data Store Read1/1 -> Product2/2
  Trigonometric Function3/1 -> Product25/1
  Add4/1 -> Out2/1
  Constant3/1 -> Add13/2

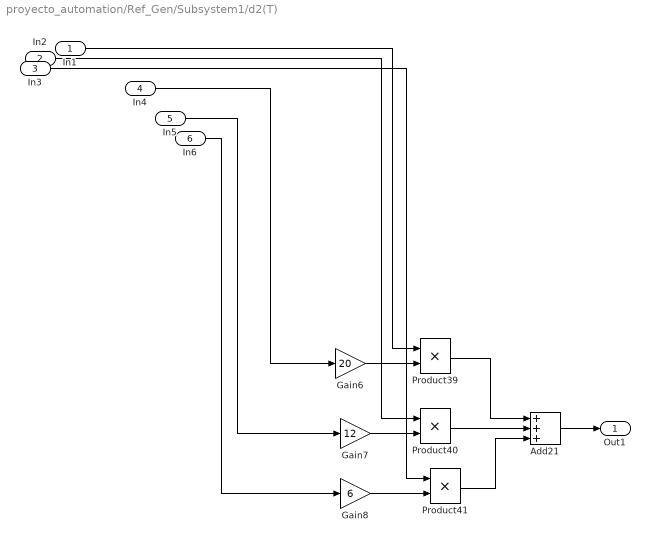
== system proyecto_automation/Ref_Gen/Subsystem1/d2(T) ==
  In1 : Inport
  In2 : Inport  Port=2
  In3 : Inport  Port=3
  In4 : Inport  Port=4
  In5 : Inport  Port=5
  In6 : Inport  Port=6
  Add21 : Sum  Inputs=+++
  Gain6 : Gain  Gain=20
  Gain7 : Gain  Gain=12
  Gain8 : Gain  Gain=6
  Product39 : Product
  Product40 : Product
  Product41 : Product
  Out1 : Outport
  wires:
  Gain7/1 -> Product40/2
  Gain8/1 -> Product41/2
  In4/1 -> Gain6/1
  In5/1 -> Gain7/1
  Gain6/1 -> Product39/2
  In6/1 -> Gain8/1
  In3/1 -> Product41/1
  In2/1 -> Product40/1
  In1/1 -> Product39/1
  Product39/1 -> Add21/1
  Product40/1 -> Add21/2
  Product41/1 -> Add21/3
  Add21/1 -> Out1/1

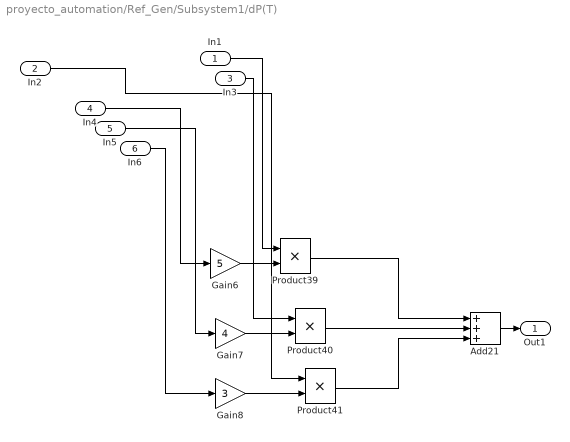
== system proyecto_automation/Ref_Gen/Subsystem1/dP(T) ==
  In1 : Inport
  In2 : Inport  Port=2
  In3 : Inport  Port=3
  In4 : Inport  Port=4
  In5 : Inport  Port=5
  In6 : Inport  Port=6
  Add21 : Sum  Inputs=+++
  Gain6 : Gain  Gain=5
  Gain7 : Gain  Gain=4
  Gain8 : Gain  Gain=3
  Product39 : Product
  Product40 : Product
  Product41 : Product
  Out1 : Outport
  wires:
  Gain8/1 -> Product41/2
  Product40/1 -> Add21/2
  In1/1 -> Product39/1
  Gain7/1 -> Product40/2
  Product41/1 -> Add21/3
  Gain6/1 -> Product39/2
  Product39/1 -> Add21/1
  In6/1 -> Gain8/1
  In5/1 -> Gain7/1
  In2/1 -> Product41/1
  Add21/1 -> Out1/1
  In4/1 -> Gain6/1
  In3/1 -> Product40/1

== system proyecto_automation/Ref_Gen/Subsystem1/Subsystem1/a ==
  In1 : Inport
  Constant1 : Constant  Value=5
  Gain4 : Gain  Gain=6
  Square2 : Math  Operator=pow  SignedPower=on  RndMeth=Zero  SaturateOnIntegerOverflow=on
  Out1 : Outport
  wires:
  Gain4/1 -> Out1/1
  In1/1 -> Square2/1
  Square2/1 -> Gain4/1
  Constant1/1 -> Square2/2

== system proyecto_automation/Ref_Gen/Subsystem1/Subsystem1/b ==
  In1 : Inport
  Constant2 : Constant  Value=4
  Gain5 : Gain  Gain=-15
  Square1 : Math  Operator=pow  SignedPower=on  RndMeth=Zero  SaturateOnIntegerOverflow=on
  Out1 : Outport
  wires:
  Constant2/1 -> Square1/2
  In1/1 -> Square1/1
  Square1/1 -> Gain5/1
  Gain5/1 -> Out1/1

== system proyecto_automation/Ref_Gen/Subsystem1/Subsystem1/c ==
  In1 : Inport
  Constant3 : Constant  Value=3
  Gain1 : Gain  Gain=10
  Square3 : Math  Operator=pow  SignedPower=on  RndMeth=Zero  SaturateOnIntegerOverflow=on
  Out1 : Outport
  wires:
  In1/1 -> Square3/1
  Constant3/1 -> Square3/2
  Square3/1 -> Gain1/1
  Gain1/1 -> Out1/1

== stateflow chart proyecto_automation/Ref_Gen/Chart1 ==
  state Line_circle_tria
    entry:
    T_1=620;
    T_2=700;
    P1x=245;
    P1y=150;
    P2x=240;
    P2y=90;
    Ppx=P2x-P1x;
    Ppy=P2y-P1y;
    Tp=T_2-T_1;
    x=1;
    y=0;
    cutting=0;
  state Line_rest_triang1
    entry:
    P1x=300;
    P1y=200;
    P2x=245;
    P2y=150;
    Ppx=P2x-P1x;
    Ppy=P2y-P1y;
    T_1=320;
    T_2=400;
    Tp=T_2-T_1;
    x=1;
    y=0;
    cutting=0;
  state a_Line_rest
    entry:
    P1x=0;
    P1y=0;
    P2x=300;
    P2y=200;
    Ppx=P2x-P1x;
    Ppy=P2y-P1y;
    T_1=0;
    T_2=320;
    Tp=T_2-T_1;
    x=1;
    y=0;
    cutting=0;
  state Circule
    entry:
    T_1=400;
    T_2=620;
    Tp=T_2-T_1;
    Gain_ce=2*pi;
    R=20;
    Pcx=225;
    Pcy=150;
    x=0;
    y=1;
    cutting=1;
  state Line_triap3_triap2
    entry:
    T_1=1130;
    T_2=1300;
    P1x=240;
    P1y=90;
    P2x=105;
    P2y=100;
    Ppx=P2x-P1x;
    Ppy=P2y-P1y;
    Tp=T_2-T_1;
    x=1;
    y=0;
    cutting=0;
  state Line_triap3_triap1
    entry:
    T_1=980;
    T_2=1130;
    P1x=120;
    P1y=50;
    P2x=240;
    P2y=90;
    Ppx=P2x-P1x;
    Ppy=P2y-P1y;
    Tp=T_2-T_1;
    x=1;
    y=0;
    cutting=1;
  state Line_triap2_triap3
    entry:
    T_1=790;
    T_2=980;
    P1x=260;
    P1y=20;
    P2x=120;
    P2y=50;
    Ppx=P2x-P1x;
    Ppy=P2y-P1y;
    Tp=T_2-T_1;
    x=1;
    y=0;
    cutting=1;
  state Line_triap1_triap2
    entry:
    T_1=700;
    T_2=790;
    P1x=240;
    P1y=90;
    P2x=260;
    P2y=20;
    Ppx=P2x-P1x;
    Ppy=P2y-P1y;
    Tp=T_2-T_1;
    x=1;
    y=0;
    cutting=1;
  state Line_triap1_triap5
    entry:
    T_1=1450;
    T_2=1600;
    P1x=45;
    P1y=100;
    P2x=105;
    P2y=100;
    Ppx=P2x-P1x;
    Ppy=P2y-P1y;
    Tp=T_2-T_1;
    x=1;
    y=0;
    cutting=1;
  state Line_triap1_triap6
    entry:
    T_1=1600;
    T_2=1900;
    P1x=105;
    P1y=100;
    P2x=300;
    P2y=200;
    Ppx=P2x-P1x;
    Ppy=P2y-P1y;
    Tp=T_2-T_1;
    x=1;
    y=0;
    cutting=0;
  state Semi_circule
    entry:
    T_1=1300;
    T_2=1450;
    Tp=T_2-T_1;
    Gain_ce=pi;
    R=30;
    Pcx=75;
    Pcy=100;
    x=0;
    y=1;
    cutting=1;
  (default) -> a_Line_rest
  Circule -> Line_circle_tria : [time>620&&time<700]
  Line_rest_triang1 -> Circule : [time>400&&time<620]
  a_Line_rest -> Line_rest_triang1 : [time>320&&time<400]
  Line_circle_tria -> Line_triap1_triap2 : [time>700&&time<790]
  Line_triap3_triap1 -> Line_triap3_triap2 : [time>1130&&time<1200]
  Line_triap2_triap3 -> Line_triap3_triap1 : [[time>980&&time<1130]]
  Line_triap1_triap2 -> Line_triap2_triap3 : [[time>790&&time<980]]
  Line_triap3_triap2 -> Semi_circule : [time>1300&&time<1450]
  Line_triap1_triap5 -> Line_triap1_triap6 : [[time>1600&&time<1900]]
  Semi_circule -> Line_triap1_triap5 : [time>1450&&time<1600]
  data: time input; T_1 output; T_2 output; P1x output; P1y output; P2x output; P2y output; x output; Tp output; Ppx output; Ppy output; Gain_ce output; Pcx output; Pcy output; R output; y output; cutting output
